simulink model "Computer"  (R2023a)
settings: Solver=VariableStepDiscrete  StartTime=0.0  StopTime=inf  RelTol=1e-3  EnableMultiTasking=on
values from neighbouring files (symbols this model uses):
  RomCode = Preprocessor(RomCode, c)    [ROM.m]
undefined symbols (not defined in the file or in its folder): c, in, RomCodeBreakpoints, RomData, RomDataBreakpoints, UartDataRx, UartDataRx_Active
libraries: Miscellaneous x281, simulink_extras x66, Memory_Blocks_Lib x46, simulink x42, Word_Multiplexers_Lib x31, Decoders_Lib x30, Encoders_Lib x10, Counters_Lib x9, Bit_Multiplexers_Lib x8, Arithmetic_Operations_Lib x5, Bit_Demultiplexers_Lib x4, Garbage x1
(part 6 of 6)

== system Computer/Word_Enable30 ==
  note: Word_Enable
  Sel(1b) : Inport
  b07 : Inport  Port=2
  b06 : Inport  Port=3
  b05 : Inport  Port=4
  b04 : Inport  Port=5
  b03 : Inport  Port=6
  b02 : Inport  Port=7
  b01 : Inport  Port=8
  b00 : Inport  Port=9
  Logical Operator{1..8} (8 alike) : Logic  IconShape=distinctive  AllPortsSameDT=off  OutDataTypeStr=boolean
  "b07 " : Outport
  "b06 " : Outport  Port=2
  "b05 " : Outport  Port=3
  "b04 " : Outport  Port=4
  "b03 " : Outport  Port=5
  "b02 " : Outport  Port=6
  "b01 " : Outport  Port=7
  "b00 " : Outport  Port=8
  wires:
  Logical Operator8/1 -> "b07 "/1  "b07"
  Logical Operator3/1 -> "b02 "/1  "b02"
  Logical Operator5/1 -> "b04 "/1  "b04"
  Logical Operator1/1 -> "b01 "/1  "b01"
  Logical Operator6/1 -> "b05 "/1  "b05"
  Logical Operator2/1 -> "b00 "/1  "b00"
  Logical Operator7/1 -> "b06 "/1  "b06"
  Logical Operator4/1 -> "b03 "/1  "b03"
  b00/1 -> Logical Operator2/2
  b01/1 -> Logical Operator1/2
  b02/1 -> Logical Operator3/2
  b03/1 -> Logical Operator4/2
  b04/1 -> Logical Operator5/2
  b05/1 -> Logical Operator6/2
  b06/1 -> Logical Operator7/2
  b07/1 -> Logical Operator8/2
  Sel(1b)/1 -> Logical Operator8/1, Logical Operator7/1, Logical Operator6/1, Logical Operator5/1, Logical Operator4/1, Logical Operator3/1, Logical Operator1/1, Logical Operator2/1

== system Computer/Word_Enable32 ==
  note: Word_Enable
  Sel(1b) : Inport
  b07 : Inport  Port=2
  b06 : Inport  Port=3
  b05 : Inport  Port=4
  b04 : Inport  Port=5
  b03 : Inport  Port=6
  b02 : Inport  Port=7
  b01 : Inport  Port=8
  b00 : Inport  Port=9
  Logical Operator{1..8} (8 alike) : Logic  IconShape=distinctive  AllPortsSameDT=off  OutDataTypeStr=boolean
  "b07 " : Outport
  "b06 " : Outport  Port=2
  "b05 " : Outport  Port=3
  "b04 " : Outport  Port=4
  "b03 " : Outport  Port=5
  "b02 " : Outport  Port=6
  "b01 " : Outport  Port=7
  "b00 " : Outport  Port=8
  wires:
  Logical Operator8/1 -> "b07 "/1  "b07"
  Logical Operator3/1 -> "b02 "/1  "b02"
  Logical Operator5/1 -> "b04 "/1  "b04"
  Logical Operator1/1 -> "b01 "/1  "b01"
  Logical Operator6/1 -> "b05 "/1  "b05"
  Logical Operator2/1 -> "b00 "/1  "b00"
  Logical Operator7/1 -> "b06 "/1  "b06"
  Logical Operator4/1 -> "b03 "/1  "b03"
  b00/1 -> Logical Operator2/2
  b01/1 -> Logical Operator1/2
  b02/1 -> Logical Operator3/2
  b03/1 -> Logical Operator4/2
  b04/1 -> Logical Operator5/2
  b05/1 -> Logical Operator6/2
  b06/1 -> Logical Operator7/2
  b07/1 -> Logical Operator8/2
  Sel(1b)/1 -> Logical Operator8/1, Logical Operator7/1, Logical Operator6/1, Logical Operator5/1, Logical Operator4/1, Logical Operator3/1, Logical Operator1/1, Logical Operator2/1

== system Computer/Word_Enable33 ==
  note: Word_Enable
  Sel(1b) : Inport
  b07 : Inport  Port=2
  b06 : Inport  Port=3
  b05 : Inport  Port=4
  b04 : Inport  Port=5
  b03 : Inport  Port=6
  b02 : Inport  Port=7
  b01 : Inport  Port=8
  b00 : Inport  Port=9
  Logical Operator{1..8} (8 alike) : Logic  IconShape=distinctive  AllPortsSameDT=off  OutDataTypeStr=boolean
  "b07 " : Outport
  "b06 " : Outport  Port=2
  "b05 " : Outport  Port=3
  "b04 " : Outport  Port=4
  "b03 " : Outport  Port=5
  "b02 " : Outport  Port=6
  "b01 " : Outport  Port=7
  "b00 " : Outport  Port=8
  wires:
  Logical Operator8/1 -> "b07 "/1  "b07"
  Logical Operator3/1 -> "b02 "/1  "b02"
  Logical Operator5/1 -> "b04 "/1  "b04"
  Logical Operator1/1 -> "b01 "/1  "b01"
  Logical Operator6/1 -> "b05 "/1  "b05"
  Logical Operator2/1 -> "b00 "/1  "b00"
  Logical Operator7/1 -> "b06 "/1  "b06"
  Logical Operator4/1 -> "b03 "/1  "b03"
  b00/1 -> Logical Operator2/2
  b01/1 -> Logical Operator1/2
  b02/1 -> Logical Operator3/2
  b03/1 -> Logical Operator4/2
  b04/1 -> Logical Operator5/2
  b05/1 -> Logical Operator6/2
  b06/1 -> Logical Operator7/2
  b07/1 -> Logical Operator8/2
  Sel(1b)/1 -> Logical Operator8/1, Logical Operator7/1, Logical Operator6/1, Logical Operator5/1, Logical Operator4/1, Logical Operator3/1, Logical Operator1/1, Logical Operator2/1

== system Computer/Word_Enable34 ==
  note: Word_Enable
  Sel(1b) : Inport
  b07 : Inport  Port=2
  b06 : Inport  Port=3
  b05 : Inport  Port=4
  b04 : Inport  Port=5
  b03 : Inport  Port=6
  b02 : Inport  Port=7
  b01 : Inport  Port=8
  b00 : Inport  Port=9
  Logical Operator{1..8} (8 alike) : Logic  IconShape=distinctive  AllPortsSameDT=off  OutDataTypeStr=boolean
  "b07 " : Outport
  "b06 " : Outport  Port=2
  "b05 " : Outport  Port=3
  "b04 " : Outport  Port=4
  "b03 " : Outport  Port=5
  "b02 " : Outport  Port=6
  "b01 " : Outport  Port=7
  "b00 " : Outport  Port=8
  wires:
  Logical Operator8/1 -> "b07 "/1  "b07"
  Logical Operator3/1 -> "b02 "/1  "b02"
  Logical Operator5/1 -> "b04 "/1  "b04"
  Logical Operator1/1 -> "b01 "/1  "b01"
  Logical Operator6/1 -> "b05 "/1  "b05"
  Logical Operator2/1 -> "b00 "/1  "b00"
  Logical Operator7/1 -> "b06 "/1  "b06"
  Logical Operator4/1 -> "b03 "/1  "b03"
  b00/1 -> Logical Operator2/2
  b01/1 -> Logical Operator1/2
  b02/1 -> Logical Operator3/2
  b03/1 -> Logical Operator4/2
  b04/1 -> Logical Operator5/2
  b05/1 -> Logical Operator6/2
  b06/1 -> Logical Operator7/2
  b07/1 -> Logical Operator8/2
  Sel(1b)/1 -> Logical Operator8/1, Logical Operator7/1, Logical Operator6/1, Logical Operator5/1, Logical Operator4/1, Logical Operator3/1, Logical Operator1/1, Logical Operator2/1

== system Computer/Word_Enable35 ==
  note: Word_Enable
  Sel(1b) : Inport
  b07 : Inport  Port=2
  b06 : Inport  Port=3
  b05 : Inport  Port=4
  b04 : Inport  Port=5
  b03 : Inport  Port=6
  b02 : Inport  Port=7
  b01 : Inport  Port=8
  b00 : Inport  Port=9
  Logical Operator{1..8} (8 alike) : Logic  IconShape=distinctive  AllPortsSameDT=off  OutDataTypeStr=boolean
  "b07 " : Outport
  "b06 " : Outport  Port=2
  "b05 " : Outport  Port=3
  "b04 " : Outport  Port=4
  "b03 " : Outport  Port=5
  "b02 " : Outport  Port=6
  "b01 " : Outport  Port=7
  "b00 " : Outport  Port=8
  wires:
  Logical Operator8/1 -> "b07 "/1  "b07"
  Logical Operator3/1 -> "b02 "/1  "b02"
  Logical Operator5/1 -> "b04 "/1  "b04"
  Logical Operator1/1 -> "b01 "/1  "b01"
  Logical Operator6/1 -> "b05 "/1  "b05"
  Logical Operator2/1 -> "b00 "/1  "b00"
  Logical Operator7/1 -> "b06 "/1  "b06"
  Logical Operator4/1 -> "b03 "/1  "b03"
  b00/1 -> Logical Operator2/2
  b01/1 -> Logical Operator1/2
  b02/1 -> Logical Operator3/2
  b03/1 -> Logical Operator4/2
  b04/1 -> Logical Operator5/2
  b05/1 -> Logical Operator6/2
  b06/1 -> Logical Operator7/2
  b07/1 -> Logical Operator8/2
  Sel(1b)/1 -> Logical Operator8/1, Logical Operator7/1, Logical Operator6/1, Logical Operator5/1, Logical Operator4/1, Logical Operator3/1, Logical Operator1/1, Logical Operator2/1

== system Computer/Word_Enable36 ==
  note: Word_Enable
  Sel(1b) : Inport
  b07 : Inport  Port=2
  b06 : Inport  Port=3
  b05 : Inport  Port=4
  b04 : Inport  Port=5
  b03 : Inport  Port=6
  b02 : Inport  Port=7
  b01 : Inport  Port=8
  b00 : Inport  Port=9
  Logical Operator{1..8} (8 alike) : Logic  IconShape=distinctive  AllPortsSameDT=off  OutDataTypeStr=boolean
  "b07 " : Outport
  "b06 " : Outport  Port=2
  "b05 " : Outport  Port=3
  "b04 " : Outport  Port=4
  "b03 " : Outport  Port=5
  "b02 " : Outport  Port=6
  "b01 " : Outport  Port=7
  "b00 " : Outport  Port=8
  wires:
  Logical Operator8/1 -> "b07 "/1  "b07"
  Logical Operator3/1 -> "b02 "/1  "b02"
  Logical Operator5/1 -> "b04 "/1  "b04"
  Logical Operator1/1 -> "b01 "/1  "b01"
  Logical Operator6/1 -> "b05 "/1  "b05"
  Logical Operator2/1 -> "b00 "/1  "b00"
  Logical Operator7/1 -> "b06 "/1  "b06"
  Logical Operator4/1 -> "b03 "/1  "b03"
  b00/1 -> Logical Operator2/2
  b01/1 -> Logical Operator1/2
  b02/1 -> Logical Operator3/2
  b03/1 -> Logical Operator4/2
  b04/1 -> Logical Operator5/2
  b05/1 -> Logical Operator6/2
  b06/1 -> Logical Operator7/2
  b07/1 -> Logical Operator8/2
  Sel(1b)/1 -> Logical Operator8/1, Logical Operator7/1, Logical Operator6/1, Logical Operator5/1, Logical Operator4/1, Logical Operator3/1, Logical Operator1/1, Logical Operator2/1

== matlab function Computer/Screen_40x25/MATLAB Function ==
  data: Framebuffer output uint8 size=[8*25 8*40]; CharTable input uint8 size=[8 8 256]; VideoMemory input uint8 size=1024
function Framebuffer = Video(CharTable, VideoMemory)
    VIDEO_MEM_SIZE = 1000;
    MAX_X = 40;
    MAX_Y = 25;
    CHAR_SIZE = 8;
    Framebuffer = zeros(MAX_Y*CHAR_SIZE, MAX_X*CHAR_SIZE, 'uint8');

    for (i = 1 : VIDEO_MEM_SIZE)
        y = idivide(uint16(i) - 1, uint16(MAX_X)) + 1;
        x = mod(uint16(i) - 1, uint16(MAX_X)) + 1;

        if (0 == VideoMemory(i))
            % Interpret as a space/blank character.
            ordNum = uint8(32);
        else
            ordNum = VideoMemory(i);
        end
        
        Framebuffer((CHAR_SIZE * (y - 1) + 1) : (CHAR_SIZE * (y - 1) + CHAR_SIZE),  ...
                    (CHAR_SIZE * (x - 1) + 1) : (CHAR_SIZE * (x - 1) + CHAR_SIZE))  ...
            = CharTable(:, :, ordNum);
    end
end

== matlab function Computer/MATLAB Function ==
  data: UartWrite input boolean; UartDataTx input uint8
function UartTxPin(UartWrite, UartDataTx)
    coder.extrinsic('evalin');
    coder.extrinsic('assignin');
    assignin('base', 'UartDataTx', UartDataTx);

    if (true == UartWrite)
        evalin('base', 'write(hSerialPort, UartDataTx, "uint8");');
    end
end

== matlab function Computer/MATLAB Function1 ==
  data: Reset input boolean; CLK input
% function active = Rx_Active_Latch(set, reset)
%     persistent state;
%     if isempty(state)
%         state = false;
%     end
% 
%     coder.extrinsic('evalin');
%     coder.extrinsic('assignin');
% 
%     if (true == set) && (false == reset)
%         state = true;
%     end
% 
%     if (true == reset)
%         state = false;
%         evalin('base', 'Rx_Active_Latch = false');
%         % assignin('base', 'Rx_Active_Latch', Rx_Active_Latch);
%     end
% end

function UartDataRx_Active(Reset, CLK)
    persistent prevCLK;
    if isempty(prevCLK)
        prevCLK = false;
    end

    coder.extrinsic('evalin');
    coder.extrinsic('set_param');
    coder.extrinsic('gcs');
    % 
    % if (true == in)
    %     state = true;
    % end
    % 
    if (true == Reset) && (true == prevCLK) && (false == CLK)
        evalin('base', 'UartDataRx_Active = false');
        set_param(gcs, 'SimulationCommand', 'update');
        % assignin('base', 'Rx_Active_Latch', Rx_Active_Latch);
    end

    prevCLK = CLK;
end
